simulink library "anchorTetherCtrl_ul"  (R2018b)
settings: Solver=VariableStepAuto  StartTime=0.0  StopTime=10.0  RelTol=1e-3
values from neighbouring files (symbols this model uses):
  ctrl = CTR.controller    [groundStation001_ts.m]    (also in groundStation001_ts3.m)
libraries: filteredPIDController_ul x3
settings Model: Creator=Erin B  LastModifiedBy=embeato2

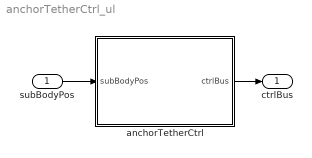
== system anchorTetherCtrl_ul ==
  subBodyPos : Inport
  anchorTetherCtrl : Subsystem
  ctrlBus : Outport  OutDataTypeStr=Bus: ctrlBus
  wires:
  subBodyPos/1 -> anchorTetherCtrl/1(subBodyPos)
  anchorTetherCtrl/1(ctrlBus) -> ctrlBus/1

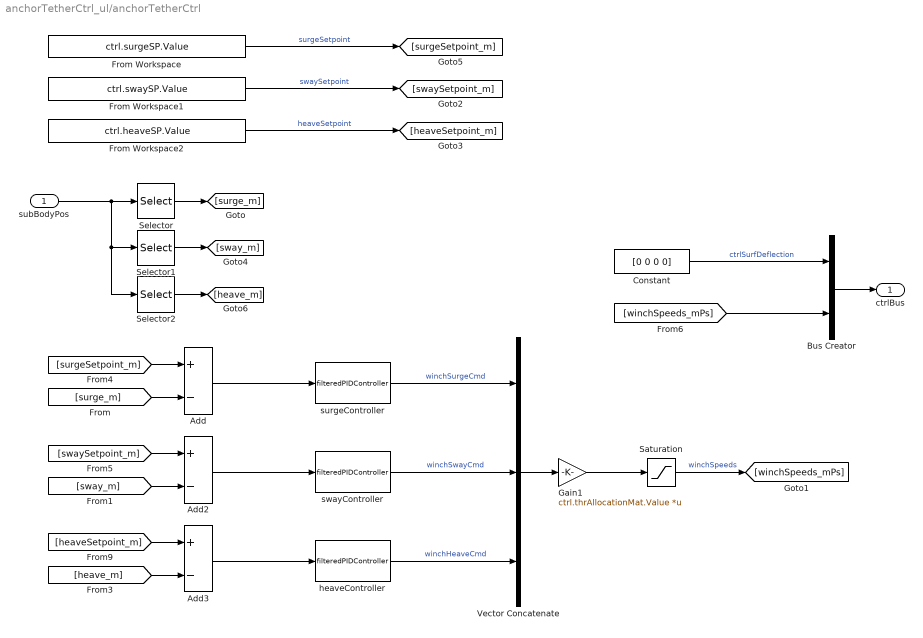
== system anchorTetherCtrl_ul/anchorTetherCtrl ==
  subBodyPos : Inport
  Add : Sum  Inputs=+-
  Add2 : Sum  Inputs=+-
  Add3 : Sum  Inputs=+-
  Bus Creator : BusCreator  Inputs=2  OutDataTypeStr=Bus: ctrlBus
  Constant : Constant  Value=[0 0 0 0]
  From Workspace : FromWorkspace  VariableName=ctrl.surgeSP.Value  SampleTime=0
  From Workspace1 : FromWorkspace  VariableName=ctrl.swaySP.Value  SampleTime=0
  From Workspace2 : FromWorkspace  VariableName=ctrl.heaveSP.Value  SampleTime=0
  Gain1 : Gain  Gain=ctrl.thrAllocationMat.Value  Multiplication=Matrix(K*u)
  Saturation : Saturate  UpperLimit=ctrl.outputSat.upperLimit.Value  LowerLimit=ctrl.outputSat.lowerLimit.Value
  Selector : Selector  InputPortWidth=3  IndexOptions=Index vector (dialog)  Indices=1  OutputSizes=1
  Selector1 : Selector  InputPortWidth=3  IndexOptions=Index vector (dialog)  Indices=2  OutputSizes=1
  Selector2 : Selector  InputPortWidth=3  IndexOptions=Index vector (dialog)  Indices=3  OutputSizes=1
  Vector Concatenate : Concatenate  NumInputs=3
  heaveController : filteredPIDController_ul/filteredPIDController  kp=ctrl.heave.kp.Value  ki=ctrl.heave.ki.Value  kd=ctrl.heave.kd.Value  Value=ctrl.heave.tau.Value
  surgeController : filteredPIDController_ul/filteredPIDController  kp=ctrl.surge.kp.Value  ki=ctrl.surge.ki.Value  kd=ctrl.surge.kd.Value  Value=ctrl.surge.tau.Value
  swayController : filteredPIDController_ul/filteredPIDController  kp=ctrl.sway.kp.Value  ki=ctrl.sway.ki.Value  kd=ctrl.sway.kd.Value  Value=ctrl.sway.tau.Value
  ctrlBus : Outport  OutDataTypeStr=Bus: ctrlBus
  wires:
  Add3/1 -> heaveController/1
  Add2/1 -> swayController/1
  [swaySetpoint_m] -> Add2/1
  From Workspace/1 -> [surgeSetpoint_m]  "surgeSetpoint"
  [heaveSetpoint_m] -> Add3/1
  Bus Creator/1 -> ctrlBus/1
  Gain1/1 -> Saturation/1
  surgeController/1 -> Vector Concatenate/1  "winchSurgeCmd"
  Add/1 -> surgeController/1
  [sway_m] -> Add2/2
  [heave_m] -> Add3/2
  heaveController/1 -> Vector Concatenate/3  "winchHeaveCmd"
  subBodyPos/1 -> Selector1/1, Selector2/1, Selector/1
  swayController/1 -> Vector Concatenate/2  "winchSwayCmd"
  [surgeSetpoint_m] -> Add/1
  Vector Concatenate/1 -> Gain1/1
  From Workspace1/1 -> [swaySetpoint_m]  "swaySetpoint"
  From Workspace2/1 -> [heaveSetpoint_m]  "heaveSetpoint"
  Selector/1 -> [surge_m]
  Selector2/1 -> [heave_m]
  Selector1/1 -> [sway_m]
  [winchSpeeds_mPs] -> Bus Creator/2
  Constant/1 -> Bus Creator/1  "ctrlSurfDeflection"
  Saturation/1 -> [winchSpeeds_mPs]  "winchSpeeds"
  [surge_m] -> Add/2
